simulink model "p1"  (R2023a)
settings: Solver=VariableStepAuto  StartTime=0.0  StopTime=10  RelTol=1e-3
settings Model: Creator=ssata  LastModifiedBy=ssata

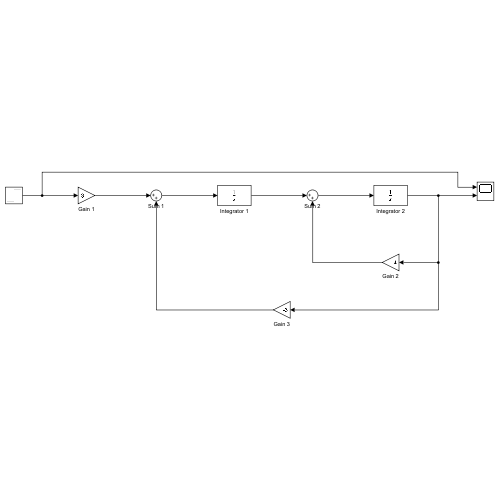
[thumbnail: Simulink's stored preview of the top-level diagram]
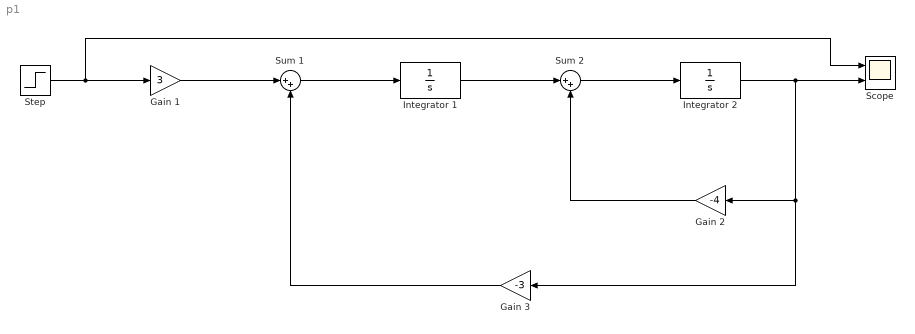
== system p1 ==
  Gain 1 : Gain  Gain=3
  Gain 2 : Gain  Gain=-4
  Gain 3 : Gain  Gain=-3
  Integrator 1 : TransferFcn  Denominator=[1 0]
  Integrator 2 : TransferFcn  Denominator=[1 0]
  Scope : Scope  NumInputPorts=2
  Step : Step  Time=0  SampleTime=0
  Sum 1 : Sum  Inputs=|++
  Sum 2 : Sum  Inputs=|++
  wires:
  Gain 1/1 -> Sum 1/1
  Sum 1/1 -> Integrator 1/1
  Integrator 1/1 -> Sum 2/1
  Gain 2/1 -> Sum 2/2
  Sum 2/1 -> Integrator 2/1
  Step/1 -> Scope/1, Gain 1/1
  Gain 3/1 -> Sum 1/2
  Integrator 2/1 -> Scope/2, Gain 3/1, Gain 2/1
